simulink model "constant_test"  (Simulink 5.0)
settings: Solver=FixedStepDiscrete  StartTime=0.0  StopTime=10.0  RelTol=1e-3
undefined symbols (not defined in the file): THREE
settings Model: Creator=sofronis  LastModifiedBy=sofronis  ExtModeAutoUpdateStatusClock=off  AlgebraicLoopMsg=error

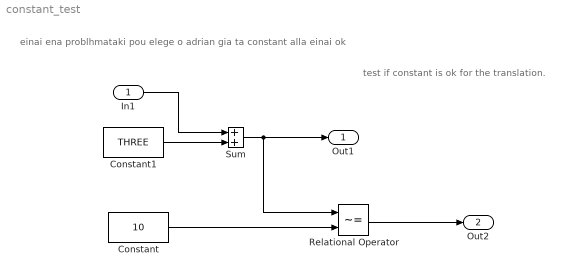
== system constant_test ==
  note: einai ena problhmataki pou elege
      | o adrian gia ta constant alla einai ok
  note: test if constant is ok for the
      | translation.
  In1 : Inport  SampleTime=1
  Constant : Constant  Value=10
  Constant1 : Constant  Value=THREE
  Relational Operator : RelationalOperator  Operator=~=  ShowAdditionalParam=on  InputSameDT=on
  Sum : Sum  SaturateOnIntegerOverflow=on  InputSameDT=on
  Out1 : Outport
  Out2 : Outport  Port=2
  wires:
  In1/1 -> Sum/1
  Sum/1 -> Out1/1, Relational Operator/1
  Constant1/1 -> Sum/2
  Constant/1 -> Relational Operator/2
  Relational Operator/1 -> Out2/1
